simulink model "lab6"  (R2023a)
settings: Solver=VariableStepDiscrete  StartTime=0.0  StopTime=26.0  RelTol=1e-3
settings Model: Creator=laura  LastModifiedBy=laura
settings OptimizationCC: ReuseModelBlockBuffer=off

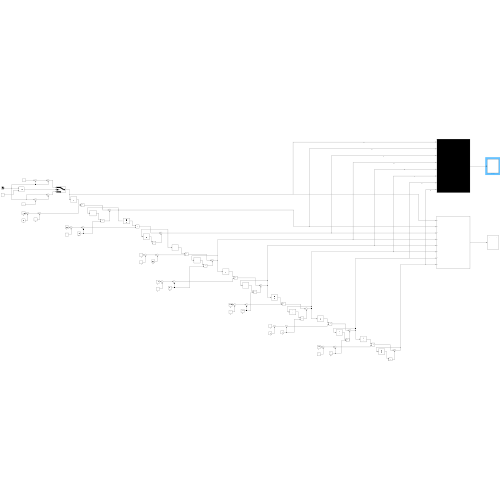
[thumbnail: Simulink's stored preview of the top-level diagram]
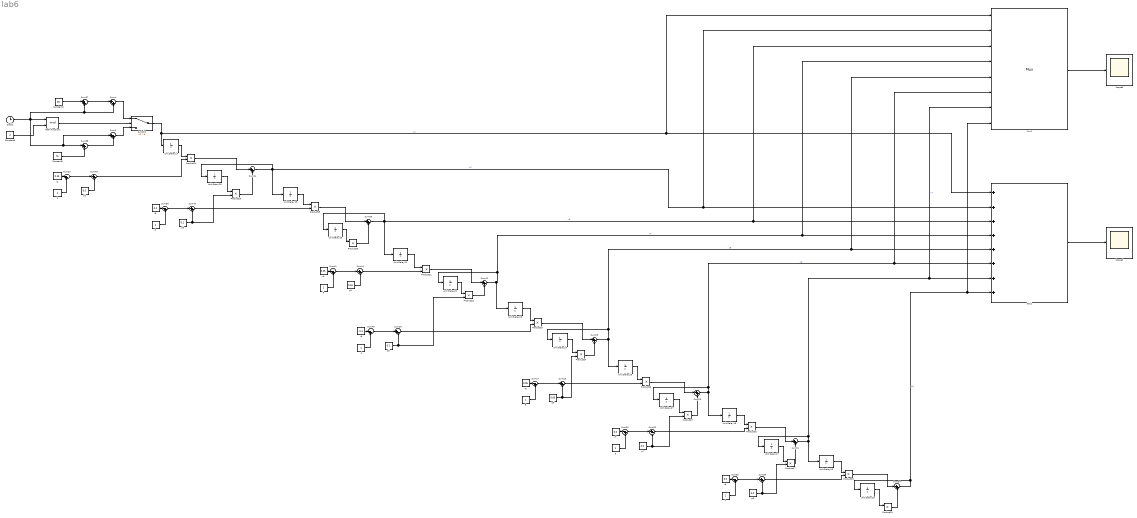
== system lab6 ==
  {1..7} (7 alike) : Constant
  Add1 : Sum  Inputs=++++++++
  Clock1 : Clock
  Constant3 : Constant  Value=2
  Constant4 : Constant  Value=30
  Constant5 : Constant  Value=70
  Math Function1 : Math  Operator=mod
  Mux1 : Mux  Inputs=8
  Product{14..27} (14 alike) : Product
  Scope2 : Scope
  Scope3 : Scope
  Sum{23,27,30,33,35,41,45} (7 alike) : Sum  Inputs=|-+
  Sum{3..4,24..25,28,31,34,37..39,42} (11 alike) : Sum  Inputs=|++
  Sum{26,29,32,36,40,43..44} (7 alike) : Sum  Inputs=|+-
  Switch1 : Switch  Criteria=u2 > Threshold  SaturateOnIntegerOverflow=off  InputSameDT=off
  Unit Delay{14..27} (14 alike) : UnitDelay  SampleTime=-1  HasFrameUpgradeWarning=on
  p2 : Constant  Value=0.0
  p3 : Constant  Value=0.1
  p4 : Constant  Value=0.15
  p5 : Constant  Value=0.1
  p6 : Constant  Value=0.05
  p7 : Constant  Value=0.0
  p8 : Constant  Value=0.0
  r2 : Constant  Value=0.15
  r3 : Constant  Value=0.2
  r4 : Constant  Value=0.25
  r5 : Constant  Value=0.1
  r6 : Constant  Value=0.05
  r7 : Constant  Value=0.0
  r8 : Constant  Value=0.0
  wires:
  Unit Delay17/1 -> Product17/1
  Sum29/1 -> Product26/2
  Unit Delay15/1 -> Product15/1
  p8/1 -> Product17/2, Sum36/2
  Sum28/1 -> Mux1/6, Add1/6, Unit Delay27/1, Unit Delay16/1  "x6"
  Unit Delay18/1 -> Product18/1
  Sum36/1 -> Product18/2
  r5/1 -> Sum45/1
  p4/1 -> Sum44/2
  Sum24/1 -> Mux1/2, Add1/2, Unit Delay15/1, Unit Delay25/1  "x2"
  Unit Delay19/1 -> Product19/1
  Sum42/1 -> Mux1/4, Add1/4, Unit Delay22/1, Unit Delay23/1  "x4"
  Sum31/1 -> Mux1/7, Add1/7, Unit Delay17/1, Unit Delay18/1  "x7"
  6/1 -> Sum30/2
  Product21/1 -> Sum42/1
  p3/1 -> Sum40/2, Product25/2
  Unit Delay24/1 -> Product24/1
  Sum35/1 -> Sum40/1
  Sum33/1 -> Sum36/1
  Unit Delay16/1 -> Product16/1
  Sum26/1 -> Product23/2
  7/1 -> Sum33/2
  Product27/1 -> Sum28/2
  Product17/1 -> Sum31/2
  Math Function1/1 -> Switch1/2
  Unit Delay21/1 -> Product21/1
  Constant3/1 -> Math Function1/2
  Sum25/1 -> Mux1/5, Add1/5, Unit Delay24/1, Unit Delay26/1  "x5"
  r8/1 -> Sum33/1
  Product25/1 -> Sum24/2
  p6/1 -> Product24/2, Sum29/2
  5/1 -> Sum27/2
  Unit Delay26/1 -> Product26/1
  r3/1 -> Sum35/1
  Constant5/1 -> Sum38/2
  p2/1 -> Sum43/2
  r7/1 -> Sum30/1
  Product14/1 -> Sum24/1
  p5/1 -> Sum26/2, Product22/2
  Product22/1 -> Sum42/2
  Unit Delay22/1 -> Product22/1
  Mux1/1 -> Scope3/1
  Sum43/1 -> Product14/2
  Add1/1 -> Scope2/1
  Constant4/1 -> Sum37/1
  Product20/1 -> Sum39/2
  r6/1 -> Sum27/1
  Product24/1 -> Sum25/2
  Clock1/1 -> Sum4/2, Sum37/2, Sum3/1, Sum38/1, Math Function1/1
  Sum41/1 -> Sum44/1
  Product26/1 -> Sum28/1
  Switch1/1 -> Mux1/1, Add1/1, Unit Delay14/1  "x1"
  Sum23/1 -> Sum43/1
  Product23/1 -> Sum25/1
  Unit Delay27/1 -> Product27/1
  Sum39/1 -> Unit Delay21/1, Mux1/3, Add1/3, Unit Delay20/1  "x3"
  Sum44/1 -> Product21/2
  Sum32/1 -> Product16/2
  1/1 -> Sum23/2
  4/1 -> Sum45/2
  Sum34/1 -> Mux1/8, Add1/8, Unit Delay19/1  "x8"
  Unit Delay20/1 -> Product20/1
  3/1 -> Sum41/2
  Sum45/1 -> Sum26/1
  Sum40/1 -> Product15/2
  r2/1 -> Sum23/1
  2/1 -> Sum35/2
  Unit Delay23/1 -> Product23/1
  Product15/1 -> Sum39/1
  Sum27/1 -> Sum29/1
  Unit Delay14/1 -> Product14/1
  Product19/1 -> Sum34/2
  Sum30/1 -> Sum32/1
  Product18/1 -> Sum34/1
  r4/1 -> Sum41/1
  p7/1 -> Sum32/2, Product27/2
  Unit Delay25/1 -> Product25/1
  Product16/1 -> Sum31/1
  Sum38/1 -> Sum3/2
  Sum37/1 -> Sum4/1
  Sum4/1 -> Switch1/1
  Sum3/1 -> Switch1/3
